simulink model "Serial_receiver"  (R2023b)
settings: Solver=FixedStepAuto  StartTime=0.0  StopTime=3  RelTol=1e-3
libraries: instrumentseriallib x2
settings Model: SimulationMode=accelerator  Creator=StevenGies  LastModifiedBy=17739
settings SolverCC: AlgebraicLoopSolver=TrustRegion
settings DebuggingCC: UnconnectedInputMsg=warning  UnconnectedOutputMsg=warning  UnconnectedLineMsg=warning
settings ModelReferenceCC: EnableRefExpFcnMdlSchedulingChecks=on

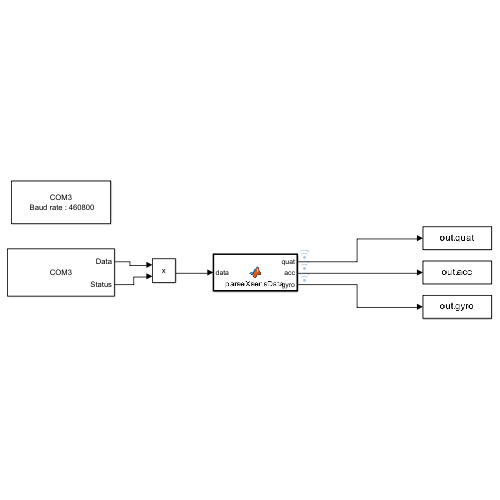
[thumbnail: Simulink's stored preview of the top-level diagram]
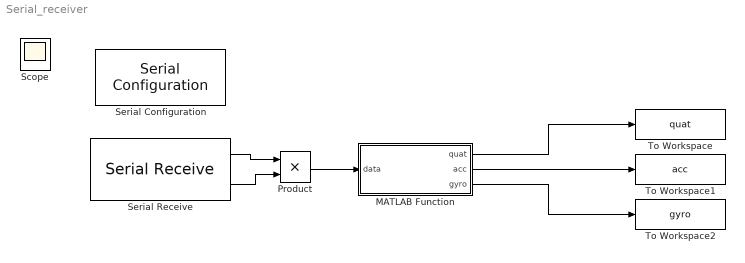
== system Serial_receiver ==
  MATLAB Function : MATLAB Function  TreatAsAtomicUnit=on
  Product : Product
  Serial Configuration : instrumentseriallib/Serial Configuration  Priority=-200000  PortSel=COM3  Port=COM3  ComPort=COM3  BaudRate=460800  DataBits=8  Parity=none  StopBits=1  ByteOrder=little-endian  FlowControl=none  Timeout=1  SimulateUsing=Interpreted execution  BlockInModel=on  aMode=1
  Serial Receive : instrumentseriallib/Serial Receive  PortSel=COM3  Port=COM3  ComPort=COM3  DataType=uint8  SaveDataType=uint8  ToggleHeader=on  Header="[ 250  255   54 ]"  DataSize=50  ToggleTerminator=on  Terminator=<none>  CustomTerminator=[]  InputFormat=Column major  ToggleDataSize=on  EnableBlockingMode=off  ActionDataUnavailable=Output custom value  ActionWhenDataUnavailable=Output custom value  CustomValue=0  SampleTime=0.0025  SimulateUsing=Interpreted execution  BlockInModel=on  aMode=1
  To Workspace : ToWorkspace  VariableName=quat  SampleTime=-1
      settings: Save2DSignal=2-D array (concatenate along first dimension)
  To Workspace1 : ToWorkspace  VariableName=acc  SampleTime=-1
      settings: Save2DSignal=2-D array (concatenate along first dimension)
  To Workspace2 : ToWorkspace  VariableName=gyro  SampleTime=-1
      settings: Save2DSignal=2-D array (concatenate along first dimension)
  Scope : Scope
  wires:
  MATLAB Function/1(quat) -> To Workspace/1
  MATLAB Function/2(acc) -> To Workspace1/1
  MATLAB Function/3(gyro) -> To Workspace2/1
  Product/1 -> MATLAB Function/1(data)
  Serial Receive/1 -> Product/1
  Serial Receive/2 -> Product/2

== matlab function Serial_receiver/MATLAB Function ==
  data: data input; quat output; acc output; gyro output
function [quat, acc, gyro]= parseXsensData(data)
% This function parses MTData2 messages. The input should be the data field
% of an MTData2 message; its header (0xFA 0xFF 0x36 or "úÿ6" should have
% already been stripped off by a preceding block. Only the most commonly
% used data fields (quaternionAngles, RateOfTurn and Acceleration) are parsed.
% MTi devices should be preconfigured (e.g. using MT Manager) to output
% these data fields. This parser can be extended for use with other data
% fields, see: https://mtidocs.xsens.com/messages

    % Initialize data outputs
    quat = typecast(uint32(zeros(4,1)),'single');
    acc = typecast(uint32(zeros(3,1)),'single');
    gyro = typecast(uint32(zeros(3,1)),'single'); 
    
    % After 0xFA 0xFF 0x36, first byte indicates the size of the message
	packetsize=data(1,1);
    
    % Checksum value can be used to confirm that a complete and valid MTData2 packet was received
    %checksum=data(packetsize+2,1);     
    
    ind = uint8(2);    
    while ind < packetsize + 1
        % Loop through the data field and check for quaternion/Acc/Gyr data
        MID = data(ind:ind+1,1);
        numbytes = data(ind+2,1);
        
        if(MID==[32; 16])           % 0x20 0x10 indicates Quaternion
            quat=parsequaternion(data(ind+3:ind+2+numbytes,1));
        elseif(MID==[128; 32])      % 0x80 0x20 indicates RateOfTurn
            gyro=parseGyr(data(ind+3:ind+2+numbytes,1));
        elseif(MID==[64; 32])       % 0x40 0x20 indicates Acceleration
            acc=parseAcc(data(ind+3:ind+2+numbytes,1));
        end
        ind = ind + 3 + numbytes;   % Increment to the next data field
     end
end

function quaternion = parsequaternion(data)
    % Parse an quaternionAngles data field, which is stored as 4x 32-bit float
    quaternion = typecast(uint32(zeros(4,1)),'single');
    hexstr = reshape(dec2hex(data)',1,32);
    quaternion(1,1) = typecast(uint32(hex2dec(hexstr(1:8))),'single');
    quaternion(2,1) = typecast(uint32(hex2dec(hexstr(9:16))),'single');
    quaternion(3,1) = typecast(uint32(hex2dec(hexstr(17:24))),'single');
    quaternion(4,1) = typecast(uint32(hex2dec(hexstr(25:32))),'single');
end

function acc = parseAcc(data)
    % Parse an Acceleration data field, which is stored as 3x 32-bit float
    acc = typecast(uint32(zeros(3,1)),'single');
    hexstr = reshape(dec2hex(data)',1,24);
    acc(1,1) = typecast(uint32(hex2dec(hexstr(1:8))),'single');
    acc(2,1) = typecast(uint32(hex2dec(hexstr(9:16))),'single');
    acc(3,1) = typecast(uint32(hex2dec(hexstr(17:24))),'single');
end

function gyr = parseGyr(data)
    % Parse a RateOfTurn data field, which is stored as 3x 32-bit float
    gyr = typecast(uint32(zeros(3,1)),'single');
    hexstr = reshape(dec2hex(data)',1,24);
    gyr(1,1) = typecast(uint32(hex2dec(hexstr(1:8))),'single');
    gyr(2,1) = typecast(uint32(hex2dec(hexstr(9:16))),'single');
    gyr(3,1) = typecast(uint32(hex2dec(hexstr(17:24))),'single');
end
